simulink model "rational_toy_to_workspace"  (R2019b)
settings: Solver=FixedStepAuto  StartTime=0.0  StopTime=20  FixedStep=0.01  RelTol=1e-3
values from neighbouring files (symbols this model uses):
  x0 = [0; 0; 0; 0; 0; 1]    [EKF_estimator.m]    (also in EKF_msd_estimator.m = [0; 0]; HAVOK.m = [0.5; 0]; KF_estimator.m = [0; 0]; Linear_regression_state_estimator.m = [0;0;0;0])
settings Model: Creator=Murray  LastModifiedBy=Murray

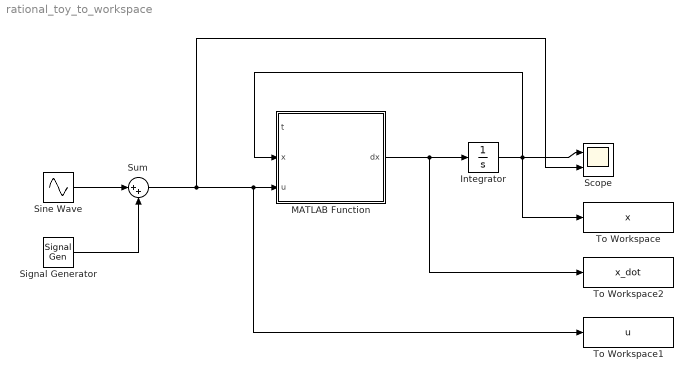
== system rational_toy_to_workspace ==
  Integrator : Integrator  InitialCondition=x0
  MATLAB Function : MATLAB Function  TreatAsAtomicUnit=on
  Scope : Scope  NumInputPorts=2
  Signal Generator : SignalGenerator  Amplitude=3  Frequency=1/2
  Sine Wave : Sin  Bias=0.5  Frequency=2*pi/5  SampleTime=0
  Sum : Sum  Inputs=|++
  To Workspace : ToWorkspace  VariableName=x  SaveFormat=Timeseries  SampleTime=-1
  To Workspace1 : ToWorkspace  VariableName=u  SaveFormat=Timeseries  SampleTime=-1
  To Workspace2 : ToWorkspace  VariableName=x_dot  SaveFormat=Timeseries  SampleTime=-1
  wires:
  MATLAB Function/1(dx) -> To Workspace2/1, Integrator/1
  Integrator/1 -> To Workspace/1, Scope/1, MATLAB Function/2(x)
  Sum/1 -> Scope/2, To Workspace1/1, MATLAB Function/3(u)
  Sine Wave/1 -> Sum/1
  Signal Generator/1 -> Sum/2

== matlab function rational_toy_to_workspace/MATLAB Function ==
  data: t input; x input; u input; dx output
function dx = rational_toy_ODE(t,x,u)
    % 2 states
    x1 = x(1,:);
    x2 = x(2,:);
    x3 = x(3,:);
    
    dx = [
            - x1 + 3*x3^3 - x2.^2 + u;
            (10*x1  - x2 - 2*x1.*x3)./(1.1 + sin(x1) + x1.^2);
            (x1.*x2 - 3*x3 + 2*x1*x2*x3)
    ];

end
